simulink model "case9"  (R2024b)
settings: Solver=FixedStepAuto  StartTime=0  StopTime=1  FixedStep=1e-7  RelTol=1e-3
values from neighbouring files (symbols this model uses):
  SG_D_1_D = 0.01056    [IEEE9_case_parameters.m]    (also in case1_parameters.m; case2_parameters.m; case3_parameters.m; case4_parameters.m)
  SG_D_1_EnableSaturation = 0    [IEEE9_case_parameters.m]    (also in case1_parameters.m; case2_parameters.m; case3_parameters.m; case4_parameters.m)
  SG_D_1_f0 = 60    [IEEE9_case_parameters.m]    (also in case1_parameters.m; case2_parameters.m; case3_parameters.m; case4_parameters.m)
  SG_D_1_H = 7.5    [IEEE9_case_parameters.m]    (also in case1_parameters.m; case2_parameters.m; case3_parameters.m; case4_parameters.m)
  SG_D_1_K_A = 20    [IEEE9_case_parameters.m]    (also in case1_parameters.m; case2_parameters.m; case3_parameters.m; case4_parameters.m)
  SG_D_1_K_E = 1.000000e+1    (= 10)    [IEEE9_case_parameters.m]    (also in case1_parameters.m; case2_parameters.m; case3_parameters.m; case4_parameters.m)
  SG_D_1_K_F = 2.363    [IEEE9_case_parameters.m]    (also in case1_parameters.m; case2_parameters.m; case3_parameters.m; case4_parameters.m)
  SG_D_1_K_s = 0.5    [IEEE9_case_parameters.m]    (also in case1_parameters.m = 5; case2_parameters.m = 5; case3_parameters.m = 5; case4_parameters.m = 5)
  SG_D_1_R_a = 0.001088    [IEEE9_case_parameters.m]    (also in case1_parameters.m; case2_parameters.m; case3_parameters.m; case4_parameters.m)
  SG_D_1_S_A = 1    [IEEE9_case_parameters.m]    (also in case1_parameters.m; case2_parameters.m; case3_parameters.m; case4_parameters.m)
  SG_D_1_S_B = 0.103    [IEEE9_case_parameters.m]    (also in case1_parameters.m; case2_parameters.m; case3_parameters.m; case4_parameters.m)
  SG_D_1_S_N = 10.659857    [IEEE9_case_parameters.m]    (also in case1_parameters.m; case2_parameters.m; case3_parameters.m; case4_parameters.m)
  SG_D_1_SpeedPara = 200    [IEEE9_case_parameters.m]    (also in case1_parameters.m; case2_parameters.m; case3_parameters.m; case4_parameters.m)
  SG_D_1_T_0 = 0.720173    [IEEE9_case_parameters.m]    (also in case1_parameters.m = 0.755522; case2_parameters.m = 0.808931; case3_parameters.m = 0.869402; case4_parameters.m = 0.729316)
  SG_D_1_T_1 = 0.3    [IEEE9_case_parameters.m]    (also in case1_parameters.m; case2_parameters.m; case3_parameters.m; case4_parameters.m)
  SG_D_1_T_2 = 0.05    [IEEE9_case_parameters.m]    (also in case1_parameters.m; case2_parameters.m; case3_parameters.m; case4_parameters.m)
  SG_D_1_T_3 = 0.02    [IEEE9_case_parameters.m]    (also in case1_parameters.m; case2_parameters.m; case3_parameters.m; case4_parameters.m)
  SG_D_1_T_4 = 0.005    [IEEE9_case_parameters.m]    (also in case1_parameters.m; case2_parameters.m; case3_parameters.m; case4_parameters.m)
  SG_D_1_T_A = 0.02    [IEEE9_case_parameters.m]    (also in case1_parameters.m; case2_parameters.m; case3_parameters.m; case4_parameters.m)
  SG_D_1_T_dd = 8.000000e+0    (= 8)    [IEEE9_case_parameters.m]    (also in case1_parameters.m; case2_parameters.m; case3_parameters.m; case4_parameters.m)
  SG_D_1_T_ddd = 0.04    [IEEE9_case_parameters.m]    (also in case1_parameters.m; case2_parameters.m; case3_parameters.m; case4_parameters.m)
  SG_D_1_T_E = 0.314    [IEEE9_case_parameters.m]    (also in case1_parameters.m; case2_parameters.m; case3_parameters.m; case4_parameters.m)
  SG_D_1_T_F = 0.35    [IEEE9_case_parameters.m]    (also in case1_parameters.m; case2_parameters.m; case3_parameters.m; case4_parameters.m)
  SG_D_1_T_qd = 0.8    [IEEE9_case_parameters.m]    (also in case1_parameters.m; case2_parameters.m; case3_parameters.m; case4_parameters.m)
  SG_D_1_T_qdd = 0.02    [IEEE9_case_parameters.m]    (also in case1_parameters.m; case2_parameters.m; case3_parameters.m; case4_parameters.m)
  SG_D_1_T_speed = 0.1    [IEEE9_case_parameters.m]    (also in case1_parameters.m = 200; case2_parameters.m = 200; case3_parameters.m = 200; case4_parameters.m = 200)
  SG_D_1_T_w = 0.5    [IEEE9_case_parameters.m]    (also in case1_parameters.m; case2_parameters.m; case3_parameters.m; case4_parameters.m)
  SG_D_1_V_ref = 1.990276    [IEEE9_case_parameters.m]    (also in case1_parameters.m = 2.042296; case2_parameters.m = 2.051388; case3_parameters.m = 2.089584; case4_parameters.m = 2.01845)
  SG_D_1_w_ref = 376.991118    [IEEE9_case_parameters.m]    (also in case1_parameters.m; case2_parameters.m; case3_parameters.m; case4_parameters.m)
  SG_D_1_wb = 6.000000e+1    (= 60)    [IEEE9_case_parameters.m]    (also in case1_parameters.m; case2_parameters.m; case3_parameters.m; case4_parameters.m)
  SG_D_1_x_d = 1.9    [IEEE9_case_parameters.m]    (also in case1_parameters.m; case2_parameters.m; case3_parameters.m; case4_parameters.m)
  SG_D_1_x_dd = 0.302    [IEEE9_case_parameters.m]    (also in case1_parameters.m; case2_parameters.m; case3_parameters.m; case4_parameters.m)
  SG_D_1_x_ddd = 0.204    [IEEE9_case_parameters.m]    (also in case1_parameters.m; case2_parameters.m; case3_parameters.m; case4_parameters.m)
  SG_D_1_x_l = 0.05    [IEEE9_case_parameters.m]    (also in case1_parameters.m; case2_parameters.m; case3_parameters.m; case4_parameters.m)
  SG_D_1_x_q = 1.3    [IEEE9_case_parameters.m]    (also in case1_parameters.m; case2_parameters.m; case3_parameters.m; case4_parameters.m)
  SG_D_1_x_qd = 0.5    [IEEE9_case_parameters.m]    (also in case1_parameters.m; case2_parameters.m; case3_parameters.m; case4_parameters.m)
  SG_D_1_x_qdd = 0.3    [IEEE9_case_parameters.m]    (also in case1_parameters.m; case2_parameters.m; case3_parameters.m; case4_parameters.m)
  SG_D_2_D = 0.02    [IEEE9_case_parameters.m]    (also in case1_parameters.m; case2_parameters.m; case3_parameters.m; case4_parameters.m)
  SG_D_2_EnableSaturation = 0    [IEEE9_case_parameters.m]    (also in case1_parameters.m; case2_parameters.m; case3_parameters.m; case4_parameters.m)
  SG_D_2_f0 = 60    [IEEE9_case_parameters.m]    (also in case1_parameters.m; case2_parameters.m; case3_parameters.m; case4_parameters.m)
  SG_D_2_H = 8.000000e+0    (= 8)    [IEEE9_case_parameters.m]    (also in case1_parameters.m; case2_parameters.m; case3_parameters.m; case4_parameters.m)
  SG_D_2_K_A = 20    [IEEE9_case_parameters.m]    (also in case1_parameters.m; case2_parameters.m; case3_parameters.m; case4_parameters.m)
  SG_D_2_K_E = 1.000000e+1    (= 10)    [IEEE9_case_parameters.m]    (also in case1_parameters.m; case2_parameters.m; case3_parameters.m; case4_parameters.m)
  SG_D_2_K_F = 2.363    [IEEE9_case_parameters.m]    (also in case1_parameters.m; case2_parameters.m; case3_parameters.m; case4_parameters.m)
  SG_D_2_K_s = 0.5    [IEEE9_case_parameters.m]    (also in case1_parameters.m = 4; case2_parameters.m = 4; case3_parameters.m = 4; case4_parameters.m = 4)
  SG_D_2_R_a = 0.001088    [IEEE9_case_parameters.m]    (also in case1_parameters.m; case2_parameters.m; case3_parameters.m; case4_parameters.m)
  SG_D_2_S_A = 1    [IEEE9_case_parameters.m]    (also in case1_parameters.m; case2_parameters.m; case3_parameters.m; case4_parameters.m)
  SG_D_2_S_B = 0.103    [IEEE9_case_parameters.m]    (also in case1_parameters.m; case2_parameters.m; case3_parameters.m; case4_parameters.m)
  SG_D_2_S_N = 10.659857    [IEEE9_case_parameters.m]    (also in case1_parameters.m; case2_parameters.m; case3_parameters.m; case4_parameters.m)
  SG_D_2_SpeedPara = 200    [IEEE9_case_parameters.m]    (also in case1_parameters.m; case2_parameters.m; case3_parameters.m; case4_parameters.m)
  SG_D_2_T_0 = 1.632913    [IEEE9_case_parameters.m]    (also in case1_parameters.m = 1.632925; case2_parameters.m = 1.632915; case3_parameters.m = 1.632914; case4_parameters.m = 1.632927)
  SG_D_2_T_1 = 0.2    [IEEE9_case_parameters.m]    (also in case1_parameters.m; case2_parameters.m; case3_parameters.m; case4_parameters.m)
  SG_D_2_T_2 = 0.05    [IEEE9_case_parameters.m]    (also in case1_parameters.m; case2_parameters.m; case3_parameters.m; case4_parameters.m)
  SG_D_2_T_3 = 0.02    [IEEE9_case_parameters.m]    (also in case1_parameters.m; case2_parameters.m; case3_parameters.m; case4_parameters.m)
  SG_D_2_T_4 = 0.005    [IEEE9_case_parameters.m]    (also in case1_parameters.m; case2_parameters.m; case3_parameters.m; case4_parameters.m)
  SG_D_2_T_A = 0.02    [IEEE9_case_parameters.m]    (also in case1_parameters.m; case2_parameters.m; case3_parameters.m; case4_parameters.m)
  SG_D_2_T_dd = 7.9    [IEEE9_case_parameters.m]    (also in case1_parameters.m; case2_parameters.m; case3_parameters.m; case4_parameters.m)
  SG_D_2_T_ddd = 0.04    [IEEE9_case_parameters.m]    (also in case1_parameters.m; case2_parameters.m; case3_parameters.m; case4_parameters.m)
  SG_D_2_T_E = 0.314    [IEEE9_case_parameters.m]    (also in case1_parameters.m; case2_parameters.m; case3_parameters.m; case4_parameters.m)
  SG_D_2_T_F = 0.35    [IEEE9_case_parameters.m]    (also in case1_parameters.m; case2_parameters.m; case3_parameters.m; case4_parameters.m)
  SG_D_2_T_qd = 0.8    [IEEE9_case_parameters.m]    (also in case1_parameters.m; case2_parameters.m; case3_parameters.m; case4_parameters.m)
  SG_D_2_T_qdd = 0.015    [IEEE9_case_parameters.m]    (also in case1_parameters.m; case2_parameters.m; case3_parameters.m; case4_parameters.m)
  SG_D_2_T_speed = 0.1    [IEEE9_case_parameters.m]    (also in case1_parameters.m = 150; case2_parameters.m = 150; case3_parameters.m = 150; case4_parameters.m = 150)
  SG_D_2_T_w = 0.35    [IEEE9_case_parameters.m]    (also in case1_parameters.m; case2_parameters.m; case3_parameters.m; case4_parameters.m)
  SG_D_2_V_ref = 2.58547    [IEEE9_case_parameters.m]    (also in case1_parameters.m = 2.597896; case2_parameters.m = 2.587136; case3_parameters.m = 2.586042; case4_parameters.m = 2.599679)
  SG_D_2_w_ref = 376.991118    [IEEE9_case_parameters.m]    (also in case1_parameters.m; case2_parameters.m; case3_parameters.m; case4_parameters.m)
  SG_D_2_wb = 6.000000e+1    (= 60)    [IEEE9_case_parameters.m]    (also in case1_parameters.m; case2_parameters.m; case3_parameters.m; case4_parameters.m)
  SG_D_2_x_d = 1.8    [IEEE9_case_parameters.m]    (also in case1_parameters.m; case2_parameters.m; case3_parameters.m; case4_parameters.m)
  SG_D_2_x_dd = 0.302    [IEEE9_case_parameters.m]    (also in case1_parameters.m; case2_parameters.m; case3_parameters.m; case4_parameters.m)
  SG_D_2_x_ddd = 0.204    [IEEE9_case_parameters.m]    (also in case1_parameters.m; case2_parameters.m; case3_parameters.m; case4_parameters.m)
  SG_D_2_x_l = 0.05    [IEEE9_case_parameters.m]    (also in case1_parameters.m; case2_parameters.m; case3_parameters.m; case4_parameters.m)
  SG_D_2_x_q = 1.25    [IEEE9_case_parameters.m]    (also in case1_parameters.m; case2_parameters.m; case3_parameters.m; case4_parameters.m)
  SG_D_2_x_qd = 0.5    [IEEE9_case_parameters.m]    (also in case1_parameters.m; case2_parameters.m; case3_parameters.m; case4_parameters.m)
  SG_D_2_x_qdd = 0.3    [IEEE9_case_parameters.m]    (also in case1_parameters.m; case2_parameters.m; case3_parameters.m; case4_parameters.m)
  SG_D_3_D = 0.02    [IEEE9_case_parameters.m]    (also in case1_parameters.m; case2_parameters.m; case3_parameters.m; case4_parameters.m)
  SG_D_3_EnableSaturation = 0    [IEEE9_case_parameters.m]    (also in case1_parameters.m; case2_parameters.m; case3_parameters.m; case4_parameters.m)
  SG_D_3_f0 = 60    [IEEE9_case_parameters.m]    (also in case1_parameters.m; case2_parameters.m; case3_parameters.m; case4_parameters.m)
  SG_D_3_H = 7.7    [IEEE9_case_parameters.m]    (also in case1_parameters.m; case2_parameters.m; case3_parameters.m; case4_parameters.m)
  SG_D_3_K_A = 20    [IEEE9_case_parameters.m]    (also in case1_parameters.m; case2_parameters.m; case3_parameters.m; case4_parameters.m)
  SG_D_3_K_E = 1.000000e+1    (= 10)    [IEEE9_case_parameters.m]    (also in case1_parameters.m; case2_parameters.m; case3_parameters.m; case4_parameters.m)
  SG_D_3_K_F = 2.363    [IEEE9_case_parameters.m]    (also in case1_parameters.m; case2_parameters.m; case3_parameters.m; case4_parameters.m)
  SG_D_3_K_s = 0.2    [IEEE9_case_parameters.m]    (also in case1_parameters.m = 2; case2_parameters.m = 2; case3_parameters.m = 2; case4_parameters.m = 2)
  SG_D_3_R_a = 0.001088    [IEEE9_case_parameters.m]    (also in case1_parameters.m; case2_parameters.m; case3_parameters.m; case4_parameters.m)
  SG_D_3_S_A = 1    [IEEE9_case_parameters.m]    (also in case1_parameters.m; case2_parameters.m; case3_parameters.m; case4_parameters.m)
  SG_D_3_S_B = 0.103    [IEEE9_case_parameters.m]    (also in case1_parameters.m; case2_parameters.m; case3_parameters.m; case4_parameters.m)
  SG_D_3_S_N = 10.659857    [IEEE9_case_parameters.m]    (also in case1_parameters.m; case2_parameters.m; case3_parameters.m; case4_parameters.m)
  SG_D_3_SpeedPara = 200    [IEEE9_case_parameters.m]    (also in case1_parameters.m; case2_parameters.m; case3_parameters.m; case4_parameters.m)
  SG_D_3_T_0 = 0.850788    [IEEE9_case_parameters.m]    (also in case1_parameters.m = 0.850786; case2_parameters.m = 0.850787; case3_parameters.m; case4_parameters.m = 0.850786)
  SG_D_3_T_1 = 0.2    [IEEE9_case_parameters.m]    (also in case1_parameters.m; case2_parameters.m; case3_parameters.m; case4_parameters.m)
  SG_D_3_T_2 = 0.05    [IEEE9_case_parameters.m]    (also in case1_parameters.m; case2_parameters.m; case3_parameters.m; case4_parameters.m)
  SG_D_3_T_3 = 0.02    [IEEE9_case_parameters.m]    (also in case1_parameters.m; case2_parameters.m; case3_parameters.m; case4_parameters.m)
  SG_D_3_T_4 = 0.005    [IEEE9_case_parameters.m]    (also in case1_parameters.m; case2_parameters.m; case3_parameters.m; case4_parameters.m)
  SG_D_3_T_A = 0.02    [IEEE9_case_parameters.m]    (also in case1_parameters.m; case2_parameters.m; case3_parameters.m; case4_parameters.m)
  SG_D_3_T_dd = 8.1    [IEEE9_case_parameters.m]    (also in case1_parameters.m; case2_parameters.m; case3_parameters.m; case4_parameters.m)
  SG_D_3_T_ddd = 0.04    [IEEE9_case_parameters.m]    (also in case1_parameters.m; case2_parameters.m; case3_parameters.m; case4_parameters.m)
  SG_D_3_T_E = 0.314    [IEEE9_case_parameters.m]    (also in case1_parameters.m; case2_parameters.m; case3_parameters.m; case4_parameters.m)
  SG_D_3_T_F = 0.35    [IEEE9_case_parameters.m]    (also in case1_parameters.m; case2_parameters.m; case3_parameters.m; case4_parameters.m)
  SG_D_3_T_qd = 0.8    [IEEE9_case_parameters.m]    (also in case1_parameters.m; case2_parameters.m; case3_parameters.m; case4_parameters.m)
  SG_D_3_T_qdd = 0.015    [IEEE9_case_parameters.m]    (also in case1_parameters.m; case2_parameters.m; case3_parameters.m; case4_parameters.m)
  SG_D_3_T_speed = 0.1    [IEEE9_case_parameters.m]    (also in case1_parameters.m = 180; case2_parameters.m = 180; case3_parameters.m = 180; case4_parameters.m = 180)
  SG_D_3_T_w = 0.4    [IEEE9_case_parameters.m]    (also in case1_parameters.m; case2_parameters.m; case3_parameters.m; case4_parameters.m)
  SG_D_3_V_ref = 1.892727    [IEEE9_case_parameters.m]    (also in case1_parameters.m = 1.906439; case2_parameters.m = 1.895535; case3_parameters.m = 1.892105; case4_parameters.m = 1.906598)
  SG_D_3_w_ref = 376.991118    [IEEE9_case_parameters.m]    (also in case1_parameters.m; case2_parameters.m; case3_parameters.m; case4_parameters.m)
  SG_D_3_wb = 6.000000e+1    (= 60)    [IEEE9_case_parameters.m]    (also in case1_parameters.m; case2_parameters.m; case3_parameters.m; case4_parameters.m)
  SG_D_3_x_d = 1.85    [IEEE9_case_parameters.m]    (also in case1_parameters.m; case2_parameters.m; case3_parameters.m; case4_parameters.m)
  SG_D_3_x_dd = 0.302    [IEEE9_case_parameters.m]    (also in case1_parameters.m; case2_parameters.m; case3_parameters.m; case4_parameters.m)
  SG_D_3_x_ddd = 0.204    [IEEE9_case_parameters.m]    (also in case1_parameters.m; case2_parameters.m; case3_parameters.m; case4_parameters.m)
  SG_D_3_x_l = 0.05    [IEEE9_case_parameters.m]    (also in case1_parameters.m; case2_parameters.m; case3_parameters.m; case4_parameters.m)
  SG_D_3_x_q = 1.2    [IEEE9_case_parameters.m]    (also in case1_parameters.m; case2_parameters.m; case3_parameters.m; case4_parameters.m)
  SG_D_3_x_qd = 0.5    [IEEE9_case_parameters.m]    (also in case1_parameters.m; case2_parameters.m; case3_parameters.m; case4_parameters.m)
  SG_D_3_x_qdd = 0.3    [IEEE9_case_parameters.m]    (also in case1_parameters.m; case2_parameters.m; case3_parameters.m; case4_parameters.m)
(part 11 of 12)

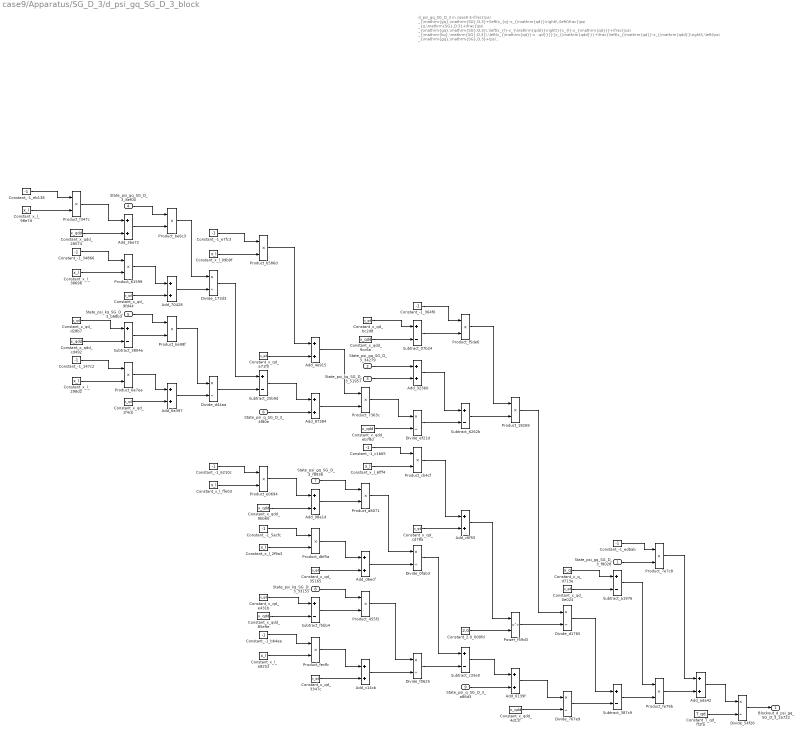
== system case9/Apparatus/SG_D_3/d_psi_gq_SG_D_3_block ==
  note: d_psi_gq_SG_D_3 in case9
      | $-\frac{\psi _{\mathrm{gq},\mathrm{SG},D,3}+\left(x_{q}-x_{\mathrm{qd}}\right)\,\left(\frac{\psi _{q,\mathrm{SG},D,3}+\frac{\psi _{\mathrm{gq},\mathrm{SG},D,3}\,\left(x_{l}-x_{\mathrm{qdd}}\right)}{x_{l}-x_{\mathrm{qd}}}+\frac{\psi _{\mathrm{kq},\mathrm{SG},D,3}\,\left(x_{\mathrm{qd}}-x_{\mathrm{qdd}}\right)}{x_{l}-x_{\mathrm{qd}}}}{x_{\mathrm{qdd}}}+\frac{\left(x_{\mathrm{qd}}-x_{\mathrm{qdd}}\right)\,\left(\psi _{\mathrm{gq},\mathrm{SG},D,3}+\psi _{\mathrm{kq},\mathrm{SG},D,3}+\frac{\left(x_{l}-x_{\mathrm{qd}}\right)\,\left(\psi _{q,\mathrm{SG},D,3}+\frac{\psi _{\mathrm{gq},\mathrm{SG},D,3}\,\left(x_{l}-x_{\mathrm{qdd}}\right)}{x_{l}-x_{\mathrm{qd}}}+\frac{\psi _{\mathrm{kq},\mathrm{SG},D,3}\,\left(x_{\mathrm{qd}}-x_{\mathrm{qdd}}\right)}{x_{l}-x_{\mathrm{qd}}}\right)}{x_{\mathrm{qdd}}}\right)}{{\left(x_{l}-x_{\mathrm{qd}}\right)}^2}\right)}{T_{\mathrm{qd}}}$
      | Automatically generated on 2025-10-31 19:35:17 .
  State_psi_gq_SG_D_3_f8028 : Inport
  State_psi_gq_SG_D_3_34279 : Inport  Port=2
  State_psi_kq_SG_D_3_51957 : Inport  Port=3
  State_psi_gq_SG_D_3_8ef00 : Inport  Port=4
  State_psi_kq_SG_D_3_b68b3 : Inport  Port=5
  State_psi_q_SG_D_3_4f80e : Inport  Port=6
  State_psi_gq_SG_D_3_f8936 : Inport  Port=7
  State_psi_kq_SG_D_3_33155 : Inport  Port=8
  State_psi_q_SG_D_3_a86d3 : Inport  Port=9
  Add_0139f : Sum
  Add_323b0 : Sum
  Add_3be72 : Sum
  Add_4e915 : Sum
  Add_6a397 : Sum
  Add_70428 : Sum
  Add_87384 : Sum
  Add_98a1d : Sum
  Add_ada42 : Sum
  Add_c14cb : Sum
  Add_c6f55 : Sum
  Add_d6ecf : Sum
  Constant_-1_147c2 : Constant  Value=-1
  Constant_-1_34866 : Constant  Value=-1
  Constant_-1_364f0 : Constant  Value=-1
  Constant_-1_5acfc : Constant  Value=-1
  Constant_-1_6210c : Constant  Value=-1
  Constant_-1_bb4ee : Constant  Value=-1
  Constant_-1_c1b65 : Constant  Value=-1
  Constant_-1_e7fc3 : Constant  Value=-1
  Constant_-1_eb138 : Constant  Value=-1
  Constant_-1_edbab : Constant  Value=-1
  Constant_2.0_000fd : Constant  Value=2.0
  Constant_T_qd_ff2fa : Constant  Value=T_qd
  Constant_x_l_09b9f : Constant  Value=x_l
  Constant_x_l_298d2 : Constant  Value=x_l
  Constant_x_l_2f9a3 : Constant  Value=x_l
  Constant_x_l_3869b : Constant  Value=x_l
  Constant_x_l_6fff4 : Constant  Value=x_l
  Constant_x_l_98e7d : Constant  Value=x_l
  Constant_x_l_a8252 : Constant  Value=x_l
  Constant_x_l_ffe03 : Constant  Value=x_l
  Constant_x_q_d713e : Constant  Value=x_q
  Constant_x_qd_0e024 : Constant  Value=x_qd
  Constant_x_qd_1f4cb : Constant  Value=x_qd
  Constant_x_qd_3347c : Constant  Value=x_qd
  Constant_x_qd_35165 : Constant  Value=x_qd
  Constant_x_qd_9fd44 : Constant  Value=x_qd
  Constant_x_qd_a71f0 : Constant  Value=x_qd
  Constant_x_qd_bc2d8 : Constant  Value=x_qd
  Constant_x_qd_cd78a : Constant  Value=x_qd
  Constant_x_qd_d28b7 : Constant  Value=x_qd
  Constant_x_qd_e431b : Constant  Value=x_qd
  Constant_x_qdd_28574 : Constant  Value=x_qdd
  Constant_x_qdd_4d11f : Constant  Value=x_qdd
  Constant_x_qdd_85e9e : Constant  Value=x_qdd
  Constant_x_qdd_9bb60 : Constant  Value=x_qdd
  Constant_x_qdd_9cc6a : Constant  Value=x_qdd
  Constant_x_qdd_cd492 : Constant  Value=x_qdd
  Constant_x_qdd_eb78d : Constant  Value=x_qdd
  Divide_0fab3 : Product  Inputs=*/
  Divide_173d3 : Product  Inputs=*/
  Divide_54f26 : Product  Inputs=*/
  Divide_767e9 : Product  Inputs=*/
  Divide_d1765 : Product  Inputs=*/
  Divide_d44aa : Product  Inputs=*/
  Divide_ef21d : Product  Inputs=*/
  Divide_f0625 : Product  Inputs=*/
  Power_f59d3 : Math  Operator=pow
  Product_18269 : Product
  Product_455f2 : Product
  Product_61599 : Product
  Product_6a7ea : Product
  Product_7363c : Product
  Product_7e7c8 : Product
  Product_a8071 : Product
  Product_b586d : Product
  Product_be6c3 : Product
  Product_be98f : Product
  Product_cb4cf : Product
  Product_dbf5a : Product
  Product_e0694 : Product
  Product_f347c : Product
  Product_f5de6 : Product
  Product_fe79b : Product
  Product_fecfb : Product
  Subtract_07b24 : Sum  Inputs=+-
  Subtract_25b9d : Sum  Inputs=+-
  Subtract_3804e : Sum  Inputs=+-
  Subtract_387c9 : Sum  Inputs=+-
  Subtract_6262b : Sum  Inputs=+-
  Subtract_a1976 : Sum  Inputs=+-
  Subtract_c33e0 : Sum  Inputs=+-
  Subtract_f5bb4 : Sum  Inputs=+-
  Blockout_d_psi_gq_SG_D_3_2a722 : Outport
  wires:
  Constant_x_l_6fff4/1 -> Product_cb4cf/2
  Constant_x_qd_d28b7/1 -> Subtract_3804e/1
  Add_4e915/1 -> Product_7363c/1
  Constant_-1_eb138/1 -> Product_f347c/1
  Add_3be72/1 -> Product_be6c3/2
  Constant_x_qdd_cd492/1 -> Subtract_3804e/2
  Constant_x_qd_a71f0/1 -> Add_4e915/2
  Constant_x_l_98e7d/1 -> Product_f347c/2
  Constant_x_l_3869b/1 -> Product_61599/2
  Add_c14cb/1 -> Divide_f0625/2
  State_psi_kq_SG_D_3_51957/1 -> Add_323b0/2
  Constant_x_qdd_28574/1 -> Add_3be72/2
  Product_f347c/1 -> Add_3be72/1
  Constant_x_qd_3347c/1 -> Add_c14cb/2
  Product_f5de6/1 -> Product_18269/1
  Constant_-1_6210c/1 -> Product_e0694/1
  Constant_-1_34866/1 -> Product_61599/1
  Constant_-1_147c2/1 -> Product_6a7ea/1
  Constant_x_l_298d2/1 -> Product_6a7ea/2
  Constant_-1_364f0/1 -> Product_f5de6/1
  Constant_-1_edbab/1 -> Product_7e7c8/1
  State_psi_gq_SG_D_3_8ef00/1 -> Product_be6c3/1
  Product_e0694/1 -> Add_98a1d/1
  Product_61599/1 -> Add_70428/1
  Product_fecfb/1 -> Add_c14cb/1
  Constant_x_qd_9fd44/1 -> Add_70428/2
  Constant_-1_5acfc/1 -> Product_dbf5a/1
  State_psi_kq_SG_D_3_b68b3/1 -> Product_be98f/1
  Subtract_3804e/1 -> Product_be98f/2
  Product_6a7ea/1 -> Add_6a397/1
  Add_98a1d/1 -> Product_a8071/2
  Add_70428/1 -> Divide_173d3/2
  Constant_x_qd_1f4cb/1 -> Add_6a397/2
  Product_be6c3/1 -> Divide_173d3/1
  Constant_T_qd_ff2fa/1 -> Divide_54f26/2
  Product_dbf5a/1 -> Add_d6ecf/1
  Product_be98f/1 -> Divide_d44aa/1
  Product_455f2/1 -> Divide_f0625/1
  Add_6a397/1 -> Divide_d44aa/2
  Constant_-1_e7fc3/1 -> Product_b586d/1
  Constant_x_qdd_eb78d/1 -> Divide_ef21d/2
  Constant_x_l_09b9f/1 -> Product_b586d/2
  Divide_173d3/1 -> Subtract_25b9d/1
  Constant_x_qd_0e024/1 -> Subtract_a1976/2
  Add_d6ecf/1 -> Divide_0fab3/2
  Divide_d44aa/1 -> Subtract_25b9d/2
  Constant_x_l_ffe03/1 -> Product_e0694/2
  Product_b586d/1 -> Add_4e915/1
  Constant_-1_c1b65/1 -> Product_cb4cf/1
  Constant_x_l_2f9a3/1 -> Product_dbf5a/2
  Subtract_25b9d/1 -> Add_87384/1
  State_psi_q_SG_D_3_4f80e/1 -> Add_87384/2
  Constant_-1_bb4ee/1 -> Product_fecfb/1
  Constant_x_qdd_9bb60/1 -> Add_98a1d/2
  Constant_x_qd_e431b/1 -> Subtract_f5bb4/1
  Constant_x_qdd_85e9e/1 -> Subtract_f5bb4/2
  Constant_x_l_a8252/1 -> Product_fecfb/2
  Add_87384/1 -> Product_7363c/2
  Constant_x_qdd_9cc6a/1 -> Subtract_07b24/2
  State_psi_gq_SG_D_3_f8936/1 -> Product_a8071/1
  Constant_x_qd_35165/1 -> Add_d6ecf/2
  Divide_d1765/1 -> Subtract_387c9/1
  State_psi_kq_SG_D_3_33155/1 -> Product_455f2/1
  Subtract_f5bb4/1 -> Product_455f2/2
  Constant_x_qd_bc2d8/1 -> Subtract_07b24/1
  State_psi_gq_SG_D_3_34279/1 -> Add_323b0/1
  Product_7363c/1 -> Divide_ef21d/1
  Product_a8071/1 -> Divide_0fab3/1
  Subtract_07b24/1 -> Product_f5de6/2
  Add_323b0/1 -> Subtract_6262b/1
  Divide_ef21d/1 -> Subtract_6262b/2
  Product_cb4cf/1 -> Add_c6f55/1
  Constant_x_qd_cd78a/1 -> Add_c6f55/2
  Divide_0fab3/1 -> Subtract_c33e0/1
  Divide_f0625/1 -> Subtract_c33e0/2
  Subtract_6262b/1 -> Product_18269/2
  Add_c6f55/1 -> Power_f59d3/1
  Constant_2.0_000fd/1 -> Power_f59d3/2
  Subtract_c33e0/1 -> Add_0139f/1
  State_psi_q_SG_D_3_a86d3/1 -> Add_0139f/2
  Product_18269/1 -> Divide_d1765/1
  Power_f59d3/1 -> Divide_d1765/2
  Add_0139f/1 -> Divide_767e9/1
  Constant_x_qdd_4d11f/1 -> Divide_767e9/2
  Constant_x_q_d713e/1 -> Subtract_a1976/1
  Divide_767e9/1 -> Subtract_387c9/2
  State_psi_gq_SG_D_3_f8028/1 -> Product_7e7c8/2
  Subtract_a1976/1 -> Product_fe79b/1
  Subtract_387c9/1 -> Product_fe79b/2
  Product_7e7c8/1 -> Add_ada42/1
  Product_fe79b/1 -> Add_ada42/2
  Add_ada42/1 -> Divide_54f26/1
  Divide_54f26/1 -> Blockout_d_psi_gq_SG_D_3_2a722/1

== system case9/Apparatus/SG_D_3/d_psi_kq_SG_D_3_block ==
  note: d_psi_kq_SG_D_3 in case9
      | $-\frac{\psi _{\mathrm{gq},\mathrm{SG},D,3}+\psi _{\mathrm{kq},\mathrm{SG},D,3}+\frac{\left(x_{l}-x_{\mathrm{qd}}\right)\,\left(\psi _{q,\mathrm{SG},D,3}+\frac{\psi _{\mathrm{gq},\mathrm{SG},D,3}\,\left(x_{l}-x_{\mathrm{qdd}}\right)}{x_{l}-x_{\mathrm{qd}}}+\frac{\psi _{\mathrm{kq},\mathrm{SG},D,3}\,\left(x_{\mathrm{qd}}-x_{\mathrm{qdd}}\right)}{x_{l}-x_{\mathrm{qd}}}\right)}{x_{\mathrm{qdd}}}}{T_{\mathrm{qdd}}}$
      | Automatically generated on 2025-10-31 19:35:18 .
  State_psi_gq_SG_D_3_74915 : Inport
  State_psi_kq_SG_D_3_5d2f2 : Inport  Port=2
  State_psi_gq_SG_D_3_703b2 : Inport  Port=3
  State_psi_kq_SG_D_3_f922d : Inport  Port=4
  State_psi_q_SG_D_3_d78bd : Inport  Port=5
  Add_31c66 : Sum
  Add_40d25 : Sum
  Add_7d483 : Sum
  Add_7fecb : Sum
  Add_82405 : Sum
  Add_980fd : Sum
  Constant_-1_21348 : Constant  Value=-1
  Constant_-1_323e6 : Constant  Value=-1
  Constant_-1_60064 : Constant  Value=-1
  Constant_-1_6904a : Constant  Value=-1
  Constant_-1_b79ad : Constant  Value=-1
  Constant_T_qdd_da107 : Constant  Value=T_qdd
  Constant_x_l_1a3a0 : Constant  Value=x_l
  Constant_x_l_81d73 : Constant  Value=x_l
  Constant_x_l_aa708 : Constant  Value=x_l
  Constant_x_l_d5787 : Constant  Value=x_l
  Constant_x_qd_3052d : Constant  Value=x_qd
  Constant_x_qd_402d2 : Constant  Value=x_qd
  Constant_x_qd_7c893 : Constant  Value=x_qd
  Constant_x_qd_b243d : Constant  Value=x_qd
  Constant_x_qdd_73ea6 : Constant  Value=x_qdd
  Constant_x_qdd_7bf6d : Constant  Value=x_qdd
  Constant_x_qdd_887ef : Constant  Value=x_qdd
  Divide_6013e : Product  Inputs=*/
  Divide_65b40 : Product  Inputs=*/
  Divide_ba257 : Product  Inputs=*/
  Divide_e09c0 : Product  Inputs=*/
  Product_04978 : Product
  Product_22e8a : Product
  Product_24c78 : Product
  Product_53787 : Product
  Product_7d090 : Product
  Product_7eb22 : Product
  Product_83074 : Product
  Product_ee610 : Product
  Subtract_178cb : Sum  Inputs=+-
  Subtract_1d2bf : Sum  Inputs=+-
  Subtract_2cb2d : Sum  Inputs=+-
  Blockout_d_psi_kq_SG_D_3_3a3de : Outport
  wires:
  State_psi_q_SG_D_3_d78bd/1 -> Add_40d25/2
  Constant_-1_21348/1 -> Product_7d090/1
  Constant_-1_60064/1 -> Product_22e8a/1
  Constant_-1_b79ad/1 -> Product_04978/1
  Constant_x_l_aa708/1 -> Product_7d090/2
  Constant_x_qdd_7bf6d/1 -> Add_82405/2
  Product_7eb22/1 -> Add_7d483/1
  Constant_x_l_81d73/1 -> Product_22e8a/2
  Constant_x_qd_3052d/1 -> Subtract_1d2bf/1
  Product_22e8a/1 -> Add_82405/1
  Constant_x_l_d5787/1 -> Product_53787/2
  Constant_x_qdd_73ea6/1 -> Subtract_1d2bf/2
  Constant_-1_6904a/1 -> Product_7eb22/1
  Constant_x_l_1a3a0/1 -> Product_7eb22/2
  State_psi_gq_SG_D_3_703b2/1 -> Product_83074/1
  Add_82405/1 -> Product_83074/2
  Add_40d25/1 -> Product_24c78/2
  Product_7d090/1 -> Add_31c66/1
  Constant_x_qd_7c893/1 -> Add_31c66/2
  State_psi_kq_SG_D_3_f922d/1 -> Product_ee610/1
  Subtract_1d2bf/1 -> Product_ee610/2
  Add_31c66/1 -> Divide_e09c0/2
  Constant_x_qd_402d2/1 -> Add_7d483/2
  Product_83074/1 -> Divide_e09c0/1
  Product_ee610/1 -> Divide_6013e/1
  Add_7d483/1 -> Divide_6013e/2
  Constant_-1_323e6/1 -> Product_53787/1
  Divide_e09c0/1 -> Subtract_2cb2d/1
  Add_7fecb/1 -> Divide_65b40/1
  Divide_6013e/1 -> Subtract_2cb2d/2
  Divide_65b40/1 -> Blockout_d_psi_kq_SG_D_3_3a3de/1
  Product_53787/1 -> Add_980fd/1
  Constant_x_qd_b243d/1 -> Add_980fd/2
  Subtract_2cb2d/1 -> Add_40d25/1
  State_psi_gq_SG_D_3_74915/1 -> Product_04978/2
  Add_980fd/1 -> Product_24c78/1
  Constant_T_qdd_da107/1 -> Divide_65b40/2
  Product_04978/1 -> Subtract_178cb/1
  State_psi_kq_SG_D_3_5d2f2/1 -> Subtract_178cb/2
  Product_24c78/1 -> Divide_ba257/1
  Constant_x_qdd_887ef/1 -> Divide_ba257/2
  Subtract_178cb/1 -> Add_7fecb/1
  Divide_ba257/1 -> Add_7fecb/2

== system case9/Apparatus/SG_D_3/d_psi_q_SG_D_3_block ==
  note: d_psi_q_SG_D_3 in case9
      | $2\,\pi \,f_{0}\,\left(v_{d,\mathrm{SG},D,3}\,\cos\left(\theta _{\mathrm{SG},D,3}\right)+v_{q,\mathrm{SG},D,3}\,\sin\left(\theta _{\mathrm{SG},D,3}\right)-\frac{R_{a}\,\left(\psi _{q,\mathrm{SG},D,3}+\frac{\psi _{\mathrm{gq},\mathrm{SG},D,3}\,\left(x_{l}-x_{\mathrm{qdd}}\right)}{x_{l}-x_{\mathrm{qd}}}+\frac{\psi _{\mathrm{kq},\mathrm{SG},D,3}\,\left(x_{\mathrm{qd}}-x_{\mathrm{qdd}}\right)}{x_{l}-x_{\mathrm{qd}}}\right)}{x_{\mathrm{qdd}}}-\frac{\psi _{d,\mathrm{SG},D,3}\,w_{\mathrm{SG},D,3}}{2\,f_{0}\,\pi }\right)$
      | Automatically generated on 2025-10-31 19:35:13 .
  State_psi_gq_SG_D_3_c1a40 : Inport
  State_psi_kq_SG_D_3_4ab7b : Inport  Port=2
  State_psi_q_SG_D_3_a8fac : Inport  Port=3
  Input_v_d_SG_D_3_2a05d : Inport  Port=4
  State_theta_SG_D_3_63669 : Inport  Port=5
  Input_v_q_SG_D_3_80c7a : Inport  Port=6
  State_theta_SG_D_3_9455b : Inport  Port=7
  State_psi_d_SG_D_3_2fcfd : Inport  Port=8
  State_w_SG_D_3_bc7af : Inport  Port=9
  Add_0468a : Sum
  Add_19c4d : Sum
  Add_6f3d3 : Sum
  Add_d83ea : Sum
  Add_da1a8 : Sum
  Constant_-1_2f120 : Constant  Value=-1
  Constant_-1_305e9 : Constant  Value=-1
  Constant_-1_b90cf : Constant  Value=-1
  Constant_-2.0_49d53 : Constant  Value=-2.0
  Constant_2.0_8dd83 : Constant  Value=2.0
  Constant_R_a_dcd83 : Constant  Value=R_a
  Constant_f0_46c84 : Constant  Value=f0
  Constant_f0_573da : Constant  Value=f0
  Constant_pi_b1c92 : Constant  Value=pi
  Constant_pi_bb7b3 : Constant  Value=pi
  Constant_x_l_519cb : Constant  Value=x_l
  Constant_x_l_7a6b8 : Constant  Value=x_l
  Constant_x_l_f5b0b : Constant  Value=x_l
  Constant_x_qd_4ae6a : Constant  Value=x_qd
  Constant_x_qd_c8053 : Constant  Value=x_qd
  Constant_x_qd_e5d55 : Constant  Value=x_qd
  Constant_x_qdd_0ed1a : Constant  Value=x_qdd
  Constant_x_qdd_e6033 : Constant  Value=x_qdd
  Constant_x_qdd_ef1fb : Constant  Value=x_qdd
  Divide_80757 : Product  Inputs=*/
  Divide_c2435 : Product  Inputs=*/
  Divide_db647 : Product  Inputs=*/
  Divide_ddcc3 : Product  Inputs=*/
  MathFunc_cos_c7d1f : Trigonometry  Operator=cos
  MathFunc_sin_0e2df : Trigonometry
  Product_1f697 : Product
  Product_21f37 : Product
  Product_27913 : Product
  Product_3d725 : Product
  Product_4db13 : Product
  Product_948bf : Product
  Product_a1836 : Product
  Product_b9784 : Product
  Product_c4dff : Product
  Product_ce782 : Product
  Product_d50d8 : Product
  Product_dd70c : Product
  Product_eef3a : Product
  Product_ef3da : Product
  Subtract_3915f : Sum  Inputs=+-
  Subtract_5999f : Sum  Inputs=+-
  Subtract_88fb1 : Sum  Inputs=+-
  Subtract_95028 : Sum  Inputs=+-
  Blockout_d_psi_q_SG_D_3_46244 : Outport
  wires:
  Constant_x_qd_c8053/1 -> Subtract_5999f/1
  Constant_pi_b1c92/1 -> Product_eef3a/2
  Product_4db13/1 -> Divide_db647/1
  Constant_x_l_519cb/1 -> Product_a1836/2
  Constant_f0_46c84/1 -> Product_dd70c/2
  State_w_SG_D_3_bc7af/1 -> Product_ce782/2
  Constant_-1_2f120/1 -> Product_b9784/1
  Constant_x_qdd_e6033/1 -> Add_19c4d/2
  Input_v_d_SG_D_3_2a05d/1 -> Product_21f37/1
  Constant_x_qdd_0ed1a/1 -> Subtract_5999f/2
  Constant_x_l_f5b0b/1 -> Product_b9784/2
  Divide_c2435/1 -> Add_d83ea/2
  Product_b9784/1 -> Add_19c4d/1
  Constant_2.0_8dd83/1 -> Product_eef3a/1
  Add_0468a/1 -> Product_4db13/2
  Constant_-1_305e9/1 -> Product_a1836/1
  Constant_x_qd_e5d55/1 -> Add_6f3d3/2
  Constant_-1_b90cf/1 -> Product_1f697/1
  Subtract_95028/1 -> Subtract_88fb1/1
  Constant_x_l_7a6b8/1 -> Product_1f697/2
  Subtract_88fb1/1 -> Add_d83ea/1
  Constant_f0_573da/1 -> Product_c4dff/2
  State_theta_SG_D_3_9455b/1 -> MathFunc_sin_0e2df/1
  Constant_x_qd_4ae6a/1 -> Add_da1a8/2
  State_psi_gq_SG_D_3_c1a40/1 -> Product_27913/1
  Add_19c4d/1 -> Product_27913/2
  Product_eef3a/1 -> Product_c4dff/1
  Product_a1836/1 -> Add_da1a8/1
  State_psi_kq_SG_D_3_4ab7b/1 -> Product_d50d8/1
  Subtract_5999f/1 -> Product_d50d8/2
  Product_1f697/1 -> Add_6f3d3/1
  MathFunc_sin_0e2df/1 -> Product_3d725/2
  Product_27913/1 -> Divide_80757/1
  Product_c4dff/1 -> Divide_c2435/2
  Add_da1a8/1 -> Divide_80757/2
  Product_d50d8/1 -> Divide_ddcc3/1
  Add_6f3d3/1 -> Divide_ddcc3/2
  Input_v_q_SG_D_3_80c7a/1 -> Product_3d725/1
  Divide_80757/1 -> Subtract_3915f/1
  Subtract_3915f/1 -> Add_0468a/1
  Divide_ddcc3/1 -> Subtract_3915f/2
  Divide_db647/1 -> Subtract_95028/1
  State_psi_q_SG_D_3_a8fac/1 -> Add_0468a/2
  Product_3d725/1 -> Subtract_88fb1/2
  Constant_R_a_dcd83/1 -> Product_4db13/1
  State_theta_SG_D_3_63669/1 -> MathFunc_cos_c7d1f/1
  Constant_x_qdd_ef1fb/1 -> Divide_db647/2
  MathFunc_cos_c7d1f/1 -> Product_21f37/2
  Constant_-2.0_49d53/1 -> Product_ef3da/1
  Product_21f37/1 -> Subtract_95028/2
  State_psi_d_SG_D_3_2fcfd/1 -> Product_ce782/1
  Constant_pi_bb7b3/1 -> Product_ef3da/2
  Product_ce782/1 -> Divide_c2435/1
  Product_ef3da/1 -> Product_dd70c/1
  Product_dd70c/1 -> Product_948bf/1
  Add_d83ea/1 -> Product_948bf/2
  Product_948bf/1 -> Blockout_d_psi_q_SG_D_3_46244/1

== system case9/Apparatus/SG_D_3/d_theta_SG_D_3_block ==
  note: d_theta_SG_D_3 in case9
      | $w_{\mathrm{SG},D,3}-2\,\pi \,f_{0}$
      | Automatically generated on 2025-10-31 19:35:20 .
  State_w_SG_D_3_18544 : Inport
  Add_4246b : Sum
  Constant_-2.0_92150 : Constant  Value=-2.0
  Constant_f0_6a4df : Constant  Value=f0
  Constant_pi_09a15 : Constant  Value=pi
  Product_96d6f : Product
  Product_e5e8d : Product
  Blockout_d_theta_SG_D_3_cb8c0 : Outport
  wires:
  Constant_-2.0_92150/1 -> Product_e5e8d/1
  Constant_pi_09a15/1 -> Product_e5e8d/2
  State_w_SG_D_3_18544/1 -> Add_4246b/2
  Product_e5e8d/1 -> Product_96d6f/1
  Constant_f0_6a4df/1 -> Product_96d6f/2
  Product_96d6f/1 -> Add_4246b/1
  Add_4246b/1 -> Blockout_d_theta_SG_D_3_cb8c0/1

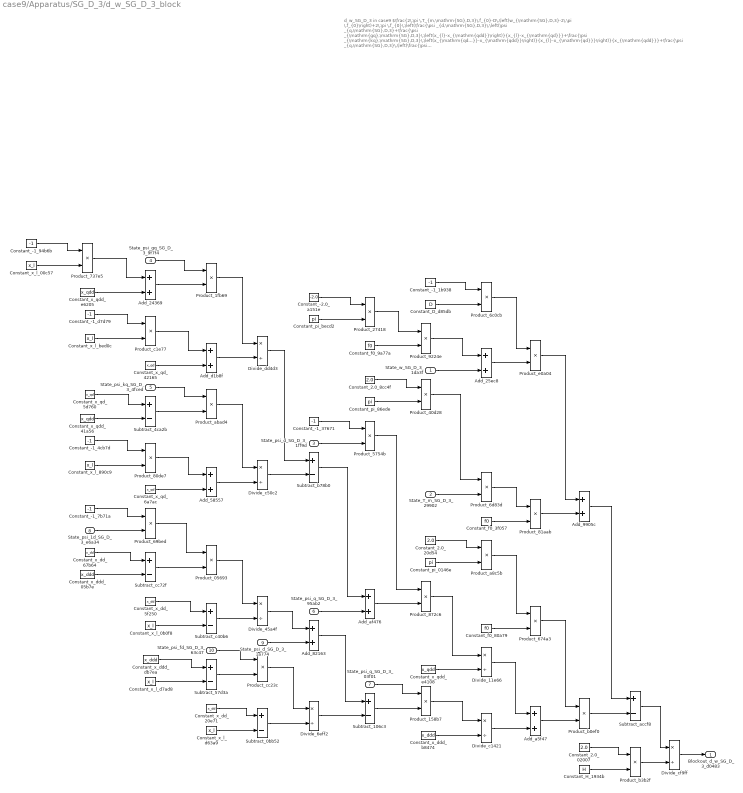
== system case9/Apparatus/SG_D_3/d_w_SG_D_3_block ==
  note: d_w_SG_D_3 in case9
      | $\frac{2\,\pi \,T_{m,\mathrm{SG},D,3}\,f_{0}-D\,\left(w_{\mathrm{SG},D,3}-2\,\pi \,f_{0}\right)+2\,\pi \,f_{0}\,\left(\frac{\psi _{d,\mathrm{SG},D,3}\,\left(\psi _{q,\mathrm{SG},D,3}+\frac{\psi _{\mathrm{gq},\mathrm{SG},D,3}\,\left(x_{l}-x_{\mathrm{qdd}}\right)}{x_{l}-x_{\mathrm{qd}}}+\frac{\psi _{\mathrm{kq},\mathrm{SG},D,3}\,\left(x_{\mathrm{qd}}-x_{\mathrm{qdd}}\right)}{x_{l}-x_{\mathrm{qd}}}\right)}{x_{\mathrm{qdd}}}+\frac{\psi _{q,\mathrm{SG},D,3}\,\left(\frac{\psi _{\mathrm{1d},\mathrm{SG},D,3}\,\left(x_{\mathrm{dd}}-x_{\mathrm{ddd}}\right)}{x_{\mathrm{dd}}-x_{l}}-\psi _{d,\mathrm{SG},D,3}+\frac{\psi _{\mathrm{fd},\mathrm{SG},D,3}\,\left(x_{\mathrm{ddd}}-x_{l}\right)}{x_{\mathrm{dd}}-x_{l}}\right)}{x_{\mathrm{ddd}}}\right)}{2\,H}$
      | Automatically generated on 2025-10-31 19:35:19 .
  State_w_SG_D_3_1da3f : Inport
  State_T_m_SG_D_3_29902 : Inport  Port=2
  State_psi_d_SG_D_3_1ff9d : Inport  Port=3
  State_psi_gq_SG_D_3_9f7f4 : Inport  Port=4
  State_psi_kq_SG_D_3_4fced : Inport  Port=5
  State_psi_q_SG_D_3_95ab2 : Inport  Port=6
  State_psi_q_SG_D_3_03f01 : Inport  Port=7
  State_psi_1d_SG_D_3_e6a34 : Inport  Port=8
  State_psi_d_SG_D_3_1a774 : Inport  Port=9
  State_psi_fd_SG_D_3_63c47 : Inport  Port=10
  Add_24369 : Sum
  Add_25ec8 : Sum
  Add_58557 : Sum
  Add_82163 : Sum
  Add_9905c : Sum
  Add_a5f47 : Sum
  Add_af476 : Sum
  Add_d1b8f : Sum
  Constant_-1_1b938 : Constant  Value=-1
  Constant_-1_37671 : Constant  Value=-1
  Constant_-1_4cb7d : Constant  Value=-1
  Constant_-1_7b71a : Constant  Value=-1
  Constant_-1_94b6b : Constant  Value=-1
  Constant_-1_d7d79 : Constant  Value=-1
  Constant_-2.0_a151e : Constant  Value=-2.0
  Constant_2.0_02007 : Constant  Value=2.0
  Constant_2.0_20d54 : Constant  Value=2.0
  Constant_2.0_8cc4f : Constant  Value=2.0
  Constant_D_d85db : Constant  Value=D
  Constant_H_1934b : Constant  Value=H
  Constant_f0_3f057 : Constant  Value=f0
  Constant_f0_80a79 : Constant  Value=f0
  Constant_f0_9a77a : Constant  Value=f0
  Constant_pi_0146e : Constant  Value=pi
  Constant_pi_86ede : Constant  Value=pi
  Constant_pi_becd2 : Constant  Value=pi
  Constant_x_dd_20e71 : Constant  Value=x_dd
  Constant_x_dd_5f250 : Constant  Value=x_dd
  Constant_x_dd_67b64 : Constant  Value=x_dd
  Constant_x_ddd_05b7e : Constant  Value=x_ddd
  Constant_x_ddd_b8474 : Constant  Value=x_ddd
  Constant_x_ddd_db7ea : Constant  Value=x_ddd
  Constant_x_l_00c57 : Constant  Value=x_l
  Constant_x_l_0b0f8 : Constant  Value=x_l
  Constant_x_l_890c9 : Constant  Value=x_l
  Constant_x_l_bed0c : Constant  Value=x_l
  Constant_x_l_d63a9 : Constant  Value=x_l
  Constant_x_l_d7ad8 : Constant  Value=x_l
  Constant_x_qd_42165 : Constant  Value=x_qd
  Constant_x_qd_5d760 : Constant  Value=x_qd
  Constant_x_qd_6a7ac : Constant  Value=x_qd
  Constant_x_qdd_41a56 : Constant  Value=x_qdd
  Constant_x_qdd_e4108 : Constant  Value=x_qdd
  Constant_x_qdd_e6205 : Constant  Value=x_qdd
  Divide_11e66 : Product  Inputs=*/
  Divide_45a4f : Product  Inputs=*/
  Divide_6eff2 : Product  Inputs=*/
  Divide_c1421 : Product  Inputs=*/
  Divide_c50c2 : Product  Inputs=*/
  Divide_cf9ff : Product  Inputs=*/
  Divide_dd4d3 : Product  Inputs=*/
  Product_05693 : Product
  Product_158b7 : Product
  Product_1fb69 : Product
  Product_27418 : Product
  Product_40d28 : Product
  Product_5754b : Product
  Product_674a3 : Product
  Product_69bed : Product
  Product_6c0cb : Product
  Product_6d83d : Product
  Product_737e5 : Product
  Product_80de7 : Product
  Product_81aab : Product
  Product_872c6 : Product
  Product_9224e : Product
  Product_a8c5b : Product
  Product_abad4 : Product
  Product_b0ef0 : Product
  Product_b3b2f : Product
  Product_c1e77 : Product
  Product_cc23c : Product
  Product_e0a04 : Product
  Subtract_0bb52 : Sum  Inputs=+-
  Subtract_106c3 : Sum  Inputs=+-
  Subtract_4ca2b : Sum  Inputs=+-
  Subtract_57d3a : Sum  Inputs=+-
  Subtract_accf8 : Sum  Inputs=+-
  Subtract_b78b0 : Sum  Inputs=+-
  Subtract_c40b6 : Sum  Inputs=+-
  Subtract_cc72f : Sum  Inputs=+-
  Blockout_d_w_SG_D_3_d0483 : Outport
  wires:
  Constant_x_qd_5d760/1 -> Subtract_4ca2b/1
  Subtract_cc72f/1 -> Product_05693/2
  Subtract_accf8/1 -> Divide_cf9ff/1
  Constant_-1_94b6b/1 -> Product_737e5/1
  Add_24369/1 -> Product_1fb69/2
  Constant_x_qdd_41a56/1 -> Subtract_4ca2b/2
  Subtract_57d3a/1 -> Product_cc23c/2
  Constant_x_l_00c57/1 -> Product_737e5/2
  State_psi_d_SG_D_3_1a774/1 -> Add_82163/2
  Add_d1b8f/1 -> Divide_dd4d3/2
  Constant_x_dd_5f250/1 -> Subtract_c40b6/1
  Constant_x_l_bed0c/1 -> Product_c1e77/2
  Constant_-1_1b938/1 -> Product_6c0cb/1
  Divide_6eff2/1 -> Subtract_106c3/2
  Constant_x_ddd_05b7e/1 -> Subtract_cc72f/2
  Constant_x_qdd_e6205/1 -> Add_24369/2
  Constant_pi_86ede/1 -> Product_40d28/2
  Product_737e5/1 -> Add_24369/1
  Constant_-2.0_a151e/1 -> Product_27418/1
  Constant_-1_d7d79/1 -> Product_c1e77/1
  Constant_2.0_20d54/1 -> Product_a8c5b/1
  Product_27418/1 -> Product_9224e/1
  Constant_-1_4cb7d/1 -> Product_80de7/1
  Subtract_b78b0/1 -> Add_af476/1
  Constant_x_l_890c9/1 -> Product_80de7/2
  Constant_x_l_d7ad8/1 -> Subtract_57d3a/2
  Constant_-1_7b71a/1 -> Product_69bed/1
  State_psi_1d_SG_D_3_e6a34/1 -> Product_69bed/2
  Constant_x_dd_67b64/1 -> Subtract_cc72f/1
  Product_69bed/1 -> Product_05693/1
  State_psi_gq_SG_D_3_9f7f4/1 -> Product_1fb69/1
  Constant_x_qd_42165/1 -> Add_d1b8f/2
  Product_c1e77/1 -> Add_d1b8f/1
  State_psi_kq_SG_D_3_4fced/1 -> Product_abad4/1
  Subtract_4ca2b/1 -> Product_abad4/2
  Product_a8c5b/1 -> Product_674a3/1
  Product_9224e/1 -> Add_25ec8/1
  Product_80de7/1 -> Add_58557/1
  State_psi_q_SG_D_3_03f01/1 -> Product_158b7/1
  Constant_x_qd_6a7ac/1 -> Add_58557/2
  Constant_x_l_0b0f8/1 -> Subtract_c40b6/2
  Constant_x_ddd_db7ea/1 -> Subtract_57d3a/1
  Constant_x_l_d63a9/1 -> Subtract_0bb52/2
  Product_1fb69/1 -> Divide_dd4d3/1
  Product_abad4/1 -> Divide_c50c2/1
  Add_58557/1 -> Divide_c50c2/2
  Product_05693/1 -> Divide_45a4f/1
  Subtract_c40b6/1 -> Divide_45a4f/2
  Constant_2.0_8cc4f/1 -> Product_40d28/1
  State_psi_fd_SG_D_3_63c47/1 -> Product_cc23c/1
  Constant_x_dd_20e71/1 -> Subtract_0bb52/1
  Divide_dd4d3/1 -> Subtract_b78b0/1
  Product_cc23c/1 -> Divide_6eff2/1
  Divide_c50c2/1 -> Subtract_b78b0/2
  Divide_45a4f/1 -> Add_82163/1
  Product_b0ef0/1 -> Subtract_accf8/2
  Subtract_0bb52/1 -> Divide_6eff2/2
  Constant_pi_becd2/1 -> Product_27418/2
  Constant_pi_0146e/1 -> Product_a8c5b/2
  Constant_-1_37671/1 -> Product_5754b/1
  State_psi_d_SG_D_3_1ff9d/1 -> Product_5754b/2
  State_psi_q_SG_D_3_95ab2/1 -> Add_af476/2
  Add_82163/1 -> Subtract_106c3/1
  Constant_f0_9a77a/1 -> Product_9224e/2
  Product_5754b/1 -> Product_872c6/1
  Add_af476/1 -> Product_872c6/2
  Subtract_106c3/1 -> Product_158b7/2
  Constant_D_d85db/1 -> Product_6c0cb/2
  State_w_SG_D_3_1da3f/1 -> Add_25ec8/2
  Product_40d28/1 -> Product_6d83d/1
  State_T_m_SG_D_3_29902/1 -> Product_6d83d/2
  Product_872c6/1 -> Divide_11e66/1
  Constant_x_qdd_e4108/1 -> Divide_11e66/2
  Product_158b7/1 -> Divide_c1421/1
  Constant_x_ddd_b8474/1 -> Divide_c1421/2
  Product_6c0cb/1 -> Product_e0a04/1
  Add_25ec8/1 -> Product_e0a04/2
  Product_6d83d/1 -> Product_81aab/1
  Constant_f0_3f057/1 -> Product_81aab/2
  Constant_f0_80a79/1 -> Product_674a3/2
  Divide_11e66/1 -> Add_a5f47/1
  Divide_c1421/1 -> Add_a5f47/2
  Product_e0a04/1 -> Add_9905c/1
  Product_81aab/1 -> Add_9905c/2
  Product_674a3/1 -> Product_b0ef0/1
  Add_a5f47/1 -> Product_b0ef0/2
  Add_9905c/1 -> Subtract_accf8/1
  Constant_2.0_02007/1 -> Product_b3b2f/1
  Constant_H_1934b/1 -> Product_b3b2f/2
  Product_b3b2f/1 -> Divide_cf9ff/2
  Divide_cf9ff/1 -> Blockout_d_w_SG_D_3_d0483/1

== system case9/Apparatus/SG_D_3/i_d_SG_D_3_block ==
  note: i_d_SG_D_3 in case9
      | $\frac{\sin\left(\theta _{\mathrm{SG},D,3}\right)\,\left(\frac{\psi _{\mathrm{1d},\mathrm{SG},D,3}\,\left(x_{\mathrm{dd}}-x_{\mathrm{ddd}}\right)}{x_{\mathrm{dd}}-x_{l}}-\psi _{d,\mathrm{SG},D,3}+\frac{\psi _{\mathrm{fd},\mathrm{SG},D,3}\,\left(x_{\mathrm{ddd}}-x_{l}\right)}{x_{\mathrm{dd}}-x_{l}}\right)}{x_{\mathrm{ddd}}}-\frac{\cos\left(\theta _{\mathrm{SG},D,3}\right)\,\left(\psi _{q,\mathrm{SG},D,3}+\frac{\psi _{\mathrm{gq},\mathrm{SG},D,3}\,\left(x_{l}-x_{\mathrm{qdd}}\right)}{x_{l}-x_{\mathrm{qd}}}+\frac{\psi _{\mathrm{kq},\mathrm{SG},D,3}\,\left(x_{\mathrm{qd}}-x_{\mathrm{qdd}}\right)}{x_{l}-x_{\mathrm{qd}}}\right)}{x_{\mathrm{qdd}}}$
      | Automatically generated on 2025-10-31 19:35:26 .
  State_psi_gq_SG_D_3_f35d9 : Inport
  State_psi_kq_SG_D_3_b0015 : Inport  Port=2
  State_psi_q_SG_D_3_4cc9d : Inport  Port=3
  State_theta_SG_D_3_cad4e : Inport  Port=4
  State_psi_1d_SG_D_3_6a382 : Inport  Port=5
  State_psi_d_SG_D_3_46ca0 : Inport  Port=6
  State_psi_fd_SG_D_3_ec227 : Inport  Port=7
  State_theta_SG_D_3_e7a7d : Inport  Port=8
  Add_0ced5 : Sum
  Add_1dc64 : Sum
  Add_2ec5a : Sum
  Add_6a173 : Sum
  Add_9d448 : Sum
  Constant_-1_0821f : Constant  Value=-1
  Constant_-1_5c58f : Constant  Value=-1
  Constant_-1_6edc3 : Constant  Value=-1
  Constant_-1_7dd96 : Constant  Value=-1
  Constant_-1_af6c3 : Constant  Value=-1
  Constant_x_dd_55b41 : Constant  Value=x_dd
  Constant_x_dd_5d8c8 : Constant  Value=x_dd
  Constant_x_dd_91407 : Constant  Value=x_dd
  Constant_x_ddd_887fb : Constant  Value=x_ddd
  Constant_x_ddd_ade8c : Constant  Value=x_ddd
  Constant_x_ddd_bcbeb : Constant  Value=x_ddd
  Constant_x_l_11c49 : Constant  Value=x_l
  Constant_x_l_5307f : Constant  Value=x_l
  Constant_x_l_5c6da : Constant  Value=x_l
  Constant_x_l_82c11 : Constant  Value=x_l
  Constant_x_l_9b151 : Constant  Value=x_l
  Constant_x_l_de47b : Constant  Value=x_l
  Constant_x_qd_85168 : Constant  Value=x_qd
  Constant_x_qd_8c4d5 : Constant  Value=x_qd
  Constant_x_qd_b48fb : Constant  Value=x_qd
  Constant_x_qdd_2ed42 : Constant  Value=x_qdd
  Constant_x_qdd_72f37 : Constant  Value=x_qdd
  Constant_x_qdd_eacdb : Constant  Value=x_qdd
  Divide_1f8f7 : Product  Inputs=*/
  Divide_2a628 : Product  Inputs=*/
  Divide_37155 : Product  Inputs=*/
  Divide_4e9d5 : Product  Inputs=*/
  Divide_720bf : Product  Inputs=*/
  Divide_fcb6b : Product  Inputs=*/
  MathFunc_cos_ab1c8 : Trigonometry  Operator=cos
  MathFunc_sin_d096c : Trigonometry
  Product_0acac : Product
  Product_0e14a : Product
  Product_29e06 : Product
  Product_34eaa : Product
  Product_48ff6 : Product
  Product_55643 : Product
  Product_85e3f : Product
  Product_e150e : Product
  Product_e400f : Product
  Product_f444b : Product
  Product_fbb8d : Product
  Subtract_38b97 : Sum  Inputs=+-
  Subtract_480ad : Sum  Inputs=+-
  Subtract_5084a : Sum  Inputs=+-
  Subtract_71e56 : Sum  Inputs=+-
  Subtract_92dde : Sum  Inputs=+-
  Subtract_d01a6 : Sum  Inputs=+-
  Subtract_d8162 : Sum  Inputs=+-
  Subtract_f7b9c : Sum  Inputs=+-
  Blockout_i_d_SG_D_3_390dd : Outport
  wires:
  Constant_x_qd_8c4d5/1 -> Subtract_f7b9c/1
  Subtract_92dde/1 -> Blockout_i_d_SG_D_3_390dd/1
  Constant_-1_0821f/1 -> Product_34eaa/1
  Constant_x_l_82c11/1 -> Product_e400f/2
  Constant_x_qdd_eacdb/1 -> Add_6a173/2
  Constant_x_qdd_2ed42/1 -> Subtract_f7b9c/2
  Constant_x_l_5307f/1 -> Product_34eaa/2
  Divide_1f8f7/1 -> Subtract_92dde/1
  Product_34eaa/1 -> Add_6a173/1
  Constant_x_ddd_bcbeb/1 -> Subtract_d8162/2
  Constant_-1_7dd96/1 -> Product_e400f/1
  Constant_-1_5c58f/1 -> Product_29e06/1
  Constant_x_l_11c49/1 -> Product_29e06/2
  State_psi_1d_SG_D_3_6a382/1 -> Product_85e3f/2
  State_psi_gq_SG_D_3_f35d9/1 -> Product_0e14a/1
  Product_85e3f/1 -> Product_55643/1
  Add_6a173/1 -> Product_0e14a/2
  Product_e400f/1 -> Add_0ced5/1
  Constant_x_qd_85168/1 -> Add_0ced5/2
  State_psi_kq_SG_D_3_b0015/1 -> Product_f444b/1
  Subtract_71e56/1 -> Divide_2a628/2
  Subtract_f7b9c/1 -> Product_f444b/2
  Product_29e06/1 -> Add_2ec5a/1
  Constant_x_ddd_ade8c/1 -> Subtract_480ad/1
  Constant_x_qd_b48fb/1 -> Add_2ec5a/2
  Constant_-1_6edc3/1 -> Product_85e3f/1
  Constant_x_dd_91407/1 -> Subtract_d8162/1
  Product_0e14a/1 -> Divide_720bf/1
  Add_0ced5/1 -> Divide_720bf/2
  Product_f444b/1 -> Divide_4e9d5/1
  Add_2ec5a/1 -> Divide_4e9d5/2
  Divide_2a628/1 -> Subtract_38b97/2
  Subtract_d8162/1 -> Product_55643/2
  State_theta_SG_D_3_cad4e/1 -> MathFunc_cos_ab1c8/1
  Constant_x_dd_55b41/1 -> Subtract_5084a/1
  Product_48ff6/1 -> Product_e150e/1
  Constant_x_l_de47b/1 -> Subtract_5084a/2
  Add_1dc64/1 -> Subtract_38b97/1
  Constant_x_l_9b151/1 -> Subtract_480ad/2
  State_theta_SG_D_3_e7a7d/1 -> MathFunc_sin_d096c/1
  Divide_720bf/1 -> Subtract_d01a6/1
  Add_9d448/1 -> Product_48ff6/2
  Divide_4e9d5/1 -> Subtract_d01a6/2
  Product_55643/1 -> Divide_37155/1
  Subtract_5084a/1 -> Divide_37155/2
  State_psi_fd_SG_D_3_ec227/1 -> Product_fbb8d/1
  Divide_fcb6b/1 -> Subtract_92dde/2
  Subtract_480ad/1 -> Product_fbb8d/2
  Constant_x_dd_5d8c8/1 -> Subtract_71e56/1
  Subtract_d01a6/1 -> Add_9d448/1
  Constant_x_l_5c6da/1 -> Subtract_71e56/2
  Constant_-1_af6c3/1 -> Product_48ff6/1
  State_psi_q_SG_D_3_4cc9d/1 -> Add_9d448/2
  Divide_37155/1 -> Add_1dc64/1
  State_psi_d_SG_D_3_46ca0/1 -> Add_1dc64/2
  Product_fbb8d/1 -> Divide_2a628/1
  MathFunc_cos_ab1c8/1 -> Product_e150e/2
  MathFunc_sin_d096c/1 -> Product_0acac/2
  Subtract_38b97/1 -> Product_0acac/1
  Product_e150e/1 -> Divide_1f8f7/1
  Constant_x_qdd_72f37/1 -> Divide_1f8f7/2
  Product_0acac/1 -> Divide_fcb6b/1
  Constant_x_ddd_887fb/1 -> Divide_fcb6b/2
